simulink model "simModel2020"  (R2023b)
settings: Solver=ode4  StartTime=0  StopTime=360  FixedStep=0.01  RelTol=1e-3
values from neighbouring files (symbols this model uses):
  B747 =     [B747.mat]
undefined symbols (not defined in the file or in its folder): airport, APP, control, Curise, Earth, env, ft, m, navData, navParam, Newton, plotTrack, Raphson, s, TakeOff, WGS84
libraries: aerolibconvert2 x18, simulink x15, sharedtransform x4, aerolibfltsims x3, aerolibatmos2 x2, shared6dof x2, aerolibasang x2, dspsrcs4 x2, aerolibwind2 x2, aerolibanimutils x1, aerolibpropulsion2 x1, aerolibtransform2 x1
(part 1 of 6)
settings Model: Creator=yansui  LastModifiedBy=30359
settings SolverCC: AlgebraicLoopSolver=TrustRegion
settings DataIOCC: SaveFormat=StructureWithTime  ReturnWorkspaceOutputs=off
settings OptimizationCC: UseDivisionForNetSlopeComputation=UseDivisionForReciprocalsOfIntegersOnly  LifeSpan=inf
settings DebuggingCC: UnderspecifiedInitializationDetection=Classic  MergeDetectMultiDrivingBlocksExec=none  UnconnectedInputMsg=warning  UnconnectedOutputMsg=warning  UnconnectedLineMsg=warning  SFExecutionAtInitializationDiag=none  ArithmeticOperatorsInVariantConditions=warning
settings HardwareCC: ProdBitPerSizeT=32  ProdBitPerPtrDiffT=32  ProdWordSize=32  ProdHWDeviceType=Specified
settings ModelReferenceCC: EnableRefExpFcnMdlSchedulingChecks=on  PropagateSignalLabelsOutOfModel=off
settings SFSimCC: CustomCodeUndefinedFunction=UseInterfaceOnly
settings RTWCC: DLArmComputeVersion=19.05
settings CodeAppCC: StateflowObjectComments=on
settings SimscapeCC: SimscapeNormalizeSystem=off

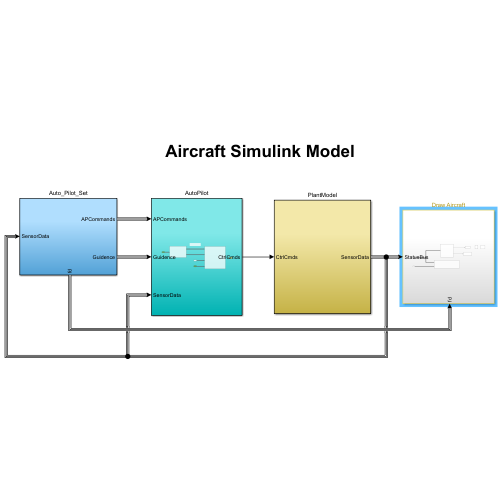
[thumbnail: Simulink's stored preview of the top-level diagram]
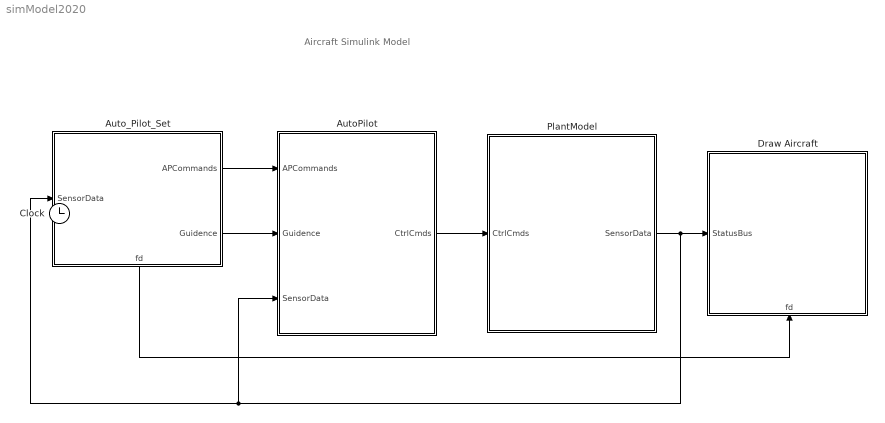
== system simModel2020 ==
  note: Aircraft Simulink Model
  AutoPilot : Subsystem
  Auto_Pilot_Set : Subsystem
      settings: PortSchema="{\"entries\":[{\"content\":{\"sides\":[{\"content\":{\"connectorIds\":[\"In1\"]},\"type\":\"ConnectorPlacement.EquallySpacedRectSide\",\"uuid\":\"ac12fa39-0519-46cb-816b-da74cf636ca7\"},{\"content\":{\"connectorIds\":[\"Out1\",\"Out2\"],\"side\":\"RIGHT\"},\"type\":\"ConnectorPlacement.EquallySpacedRectSide\",\"uuid\":\"cbf50b70-7502-46b3-9fdc-f239a08b8b7e\"},{\"content\":{\"connectorIds\":[],\"side\":\"TOP\"},\"type\":\"ConnectorPlacement.EquallySpacedRectSide\",\"uuid\":\"332bbf84-3788-4a39-9398-3a07aeea103a\"},{\"content\":{\"connectorIds\":[\"Out3\"],\"side\":\"BOTTOM\"},\"type\":\"ConnectorPlacement.EquallySpacedRectSide\",\"uuid\":\"7c0f671f-6fd4-43aa-82e5-0c8cee8639f5\"},{\"content\":{\"connectorIds\":[],\"side\":\"HIDDEN\"},\"type\":\"ConnectorPlacement.EquallySpacedRectSide\",\"uuid\":\"2f1a0ecd-686d-482d-b7d9-7339c0c9d807\"}]},\"type\":\"ConnectorPlacement.EquallySpacedConnector\",\"uuid\":\"bfc57a22-0ee0-4914-8111-1a37d4451974\"}],\"packageUris\":[\"http://schema.mathworks.com/mf0/Connector/R2020b\"],\"version\":\"1.0\"}"
  Draw Aircraft : Subsystem
      settings: PortSchema="{\"entries\":[{\"content\":{\"sides\":[{\"content\":{\"connectorIds\":[\"In1\"]},\"type\":\"ConnectorPlacement.EquallySpacedRectSide\",\"uuid\":\"f18468e1-33a6-4018-8fd5-26c86a421d63\"},{\"content\":{\"connectorIds\":[],\"side\":\"RIGHT\"},\"type\":\"ConnectorPlacement.EquallySpacedRectSide\",\"uuid\":\"f55cc71b-d18c-4aeb-b394-bdad06d8ea35\"},{\"content\":{\"connectorIds\":[],\"side\":\"TOP\"},\"type\":\"ConnectorPlacement.EquallySpacedRectSide\",\"uuid\":\"56c08431-7be0-4743-a300-4e3bf9f02124\"},{\"content\":{\"connectorIds\":[\"In2\"],\"side\":\"BOTTOM\"},\"type\":\"ConnectorPlacement.EquallySpacedRectSide\",\"uuid\":\"9c457df7-be2c-407c-bd8c-2d1e2b999c83\"},{\"content\":{\"connectorIds\":[],\"side\":\"HIDDEN\"},\"type\":\"ConnectorPlacement.EquallySpacedRectSide\",\"uuid\":\"89330191-b594-413f-b61d-27434e3fab37\"}]},\"type\":\"ConnectorPlacement.EquallySpacedConnector\",\"uuid\":\"9b92ccae-74d0-4af6-bd5d-a19e9caf359d\"}],\"packageUris\":[\"http://schema.mathworks.com/mf0/Connector/R2020b\"],\"version\":\"1.0\"}"
  PlantModel : Subsystem
  Clock : Clock
      settings: IOType=siggen
  wires:
  AutoPilot/1(CtrlCmds) -> PlantModel/1(CtrlCmds)
  Auto_Pilot_Set/2(Guidence) -> AutoPilot/2(Guidence)
  Auto_Pilot_Set/1(APCommands) -> AutoPilot/1(APCommands)
  PlantModel/1(SensorData) -> Auto_Pilot_Set/1(SensorData), AutoPilot/3(SensorData), Draw Aircraft/1(StatusBus)
  Auto_Pilot_Set/3(fd) -> Draw Aircraft/2(fd)

== system simModel2020/AutoPilot ==
  note: B747 Aircraft Controller
  APCommands : Inport
  Guidence : Inport  Port=2
  SensorData : Inport  Port=3  BusOutputAsStruct=on
  InnerLoopAutopilot : Subsystem  TreatAsAtomicUnit=on
  SensorFilter : Subsystem  TreatAsAtomicUnit=on
  CtrlCmds : Outport  BusOutputAsStruct=on
  wires:
  SensorData/1 -> SensorFilter/1(SensorData)
  SensorFilter/1(StateBus) -> InnerLoopAutopilot/1(StateBus)
  APCommands/1 -> InnerLoopAutopilot/3(APCommands)
  SensorFilter/2(Engine) -> InnerLoopAutopilot/2(Engine)
  Guidence/1 -> InnerLoopAutopilot/4(Guidence)
  InnerLoopAutopilot/1(CtrlCmds) -> CtrlCmds/1

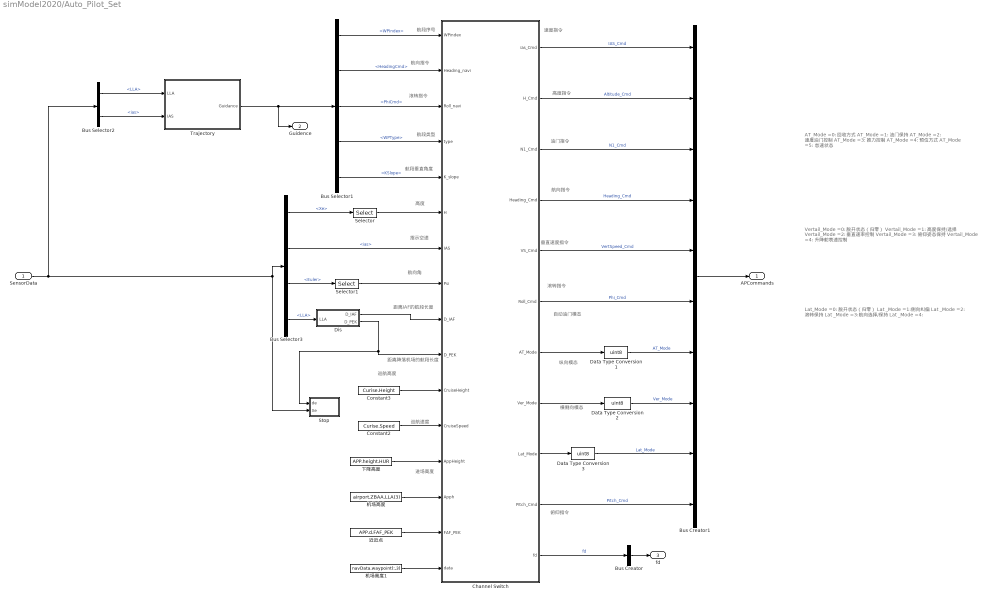
== system simModel2020/Auto_Pilot_Set ==
  note: 俯仰指令
  note: 横侧向模态
  note: 纵向模态
  note: 自动油门模态
  note: 滚转指令
  note: 垂直速度指令
  note: 航向指令
  note: 油门指令
  note: 高度指令
  note: 速度指令
  note: 航段序号
  note: 航向指令
  note: 滚转指令
  note: 航段类型
  note: 航段垂直角度
  note: 高度
  note: 指示空速
  note: 航向角
  note: 进场高度
  note: 巡航速度
  note: 巡航高度
  note: Lat_Mode =0: 脱开状态（归零）
      | Lat _Mode =1:侧向纠偏
      | Lat _Mode =2: 滚转保持
      | Lat _Mode =3:航向选择/保持
      | Lat _Mode =4:
  note: Vertail_Mode =0: 脱开状态（归零）
      | Vertail_Mode =1: 高度保持/选择
      | Vertail_Mode =2: 垂直速率控制
      | Vertail_Mode =3: 俯仰姿态保持
      | Vertail_Mode =4: 升降舵表速控制
  note: AT_Mode =0: 回收方式
      | AT_Mode =1: 油门保持
      | AT_Mode =2: 速度油门控制
      | AT_Mode =3: 推力控制
      | AT_Mode =4: 预位方式
      | AT_Mode =5: 怠速状态
  note: 距离IAF的航段长度
  note: 距离降落机场的航段长度
  SensorData : Inport
  Bus Creator : BusCreator  Inputs=1
  Bus Creator1 : BusCreator  Inputs=10
  Bus Selector1 : BusSelector  OutputSignals=WPIndex,HeadingCmd,PhiCmd,WPType,KSlope
  Bus Selector2 : BusSelector  OutputSignals=LLA,ias
  Bus Selector3 : BusSelector  OutputSignals=Xe,ias,Euler,LLA
  Channel Switch : Stateflow chart  TreatAsAtomicUnit=on
  Constant2 : Constant  Value=Curise.Speed
  Constant3 : Constant  Value=Curise.Height
  Data Type Conversion1 : DataTypeConversion  OutDataTypeStr=uint8  SaturateOnIntegerOverflow=off  RndMeth=Floor
  Data Type Conversion2 : DataTypeConversion  OutDataTypeStr=uint8  SaturateOnIntegerOverflow=off  RndMeth=Floor
  Data Type Conversion3 : DataTypeConversion  OutDataTypeStr=uint8  SaturateOnIntegerOverflow=off  RndMeth=Floor
  Dis : Subsystem
  Selector : Selector  InputPortWidth=3  IndexOptions=Index vector (dialog)  Indices=[3]  OutputSizes=1
  Selector1 : Selector  InputPortWidth=3  IndexOptions=Index vector (dialog)  Indices=[3]  OutputSizes=1
  Stop : Subsystem
  Trajectory : Subsystem
  下降高度 : Constant  Value=APP.height.HUR
  机场高度 : Constant  Value=airport.ZBAA.LLA(3)
  机场高度1 : Constant  Value=navData.waypoint(:,3)
  近近点 : Constant  Value=APP.d.FAF_PEK
  APCommands : Outport
  Guidence : Outport  Port=2
  fd : Outport  Port=3
  wires:
  Channel Switch/3(N1_Cmd) -> Bus Creator1/3  "N1_Cmd"
  Channel Switch/1(ias_Cmd) -> Bus Creator1/1  "IAS_Cmd"
  Channel Switch/5(VS_Cmd) -> Bus Creator1/5  "VertSpeed_Cmd"
  Channel Switch/2(H_Cmd) -> Bus Creator1/2  "Altitude_Cmd"
  Channel Switch/4(Heading_Cmd) -> Bus Creator1/4  "Heading_Cmd"
  Channel Switch/6(Roll_Cmd) -> Bus Creator1/6  "Phi_Cmd"
  Data Type Conversion3/1 -> Bus Creator1/9  "Lat_Mode"
  Data Type Conversion2/1 -> Bus Creator1/8  "Ver_Mode"
  Data Type Conversion1/1 -> Bus Creator1/7  "AT_Mode"
  Bus Selector3/4 -> Dis/1(LLA)  "<LLA>"
  Dis/1(D_IAF) -> Channel Switch/9(D_IAF)
  Dis/2(D_PEK) -> Stop/1(de), Channel Switch/10(D_PEK)
  Constant3/1 -> Channel Switch/11(CruiseHeight)
  Constant2/1 -> Channel Switch/12(CruiseSpeed)
  下降高度/1 -> Channel Switch/13(AppHeight)
  Bus Selector3/2 -> Channel Switch/7(IAS)  "<ias>"
  Bus Selector3/1 -> Selector/1  "<Xe>"
  Selector/1 -> Channel Switch/6(H)
  Bus Creator1/1 -> APCommands/1
  SensorData/1 -> Bus Selector2/1, Stop/2(Xe), Bus Selector3/1
  Channel Switch/7(AT_Mode) -> Data Type Conversion1/1
  Channel Switch/8(Ver_Mode) -> Data Type Conversion2/1
  Channel Switch/9(Lat_Mode) -> Data Type Conversion3/1
  Trajectory/1(Guidance) -> Guidence/1, Bus Selector1/1
  Bus Selector1/2 -> Channel Switch/2(Heading_navi)  "<HeadingCmd>"
  Bus Selector1/3 -> Channel Switch/3(Roll_navi)  "<PhiCmd>"
  Bus Selector1/4 -> Channel Switch/4(type)  "<WPType>"
  Bus Selector1/5 -> Channel Switch/5(K_slope)  "<KSlope>"
  Bus Selector2/1 -> Trajectory/1(LLA)  "<LLA>"
  Bus Selector2/2 -> Trajectory/2(IAS)  "<ias>"
  Bus Selector1/1 -> Channel Switch/1(WPindex)  "<WPIndex>"
  Bus Selector3/3 -> Selector1/1  "<Euler>"
  Selector1/1 -> Channel Switch/8(Psi)
  Channel Switch/10(Pitch_Cmd) -> Bus Creator1/10  "Pitch_Cmd"
  机场高度/1 -> Channel Switch/14(Apph)
  近近点/1 -> Channel Switch/15(FAF_PEK)
  机场高度1/1 -> Channel Switch/16(data)
  Channel Switch/11(fd) -> Bus Creator/1  "fd"
  Bus Creator/1 -> fd/1

== system simModel2020/Draw Aircraft ==
  StatusBus : Inport
  fd : Inport  Port=2
  DataOut : Subsystem
  DataToFlightgear : Subsystem
  FlightGear : Subsystem
  Generate Run Script1 : aerolibfltsims/Generate Run Script  Architecture=Win64  dataFlow=Send  GeometryModelName=f15c  AirportId=ZUUU  RunwayId=20  InitialAltitude=0  InitialHeading=200  OffsetDistance=0  OffsetAzimuth=0  InstallScenery=on  DisableShaders=off  OriginAddress=127.0.0.1  DestinationPort=5502  OriginPort=5505  LocalAddress=127.0.0.1  OutputFileName=runfg.bat  FlightGearBaseDirectory=D:\MATLAB\FlightGear 2020.3
  Interpreted MATLAB Function1 : MATLABFcn  MATLABFcn=plotTrack(u)  OutputDimensions=0  Output1D=off
  Simulation Pace : aerolibanimutils/Simulation Pace  SimulationPace=100  SleepMode=MATLAB Thread  OutputPaceError=off  SampleTime=B747.sampleTime
      settings: AttributesFormatString=%<SimulationPace> sec/sec
  wires:
  StatusBus/1 -> DataToFlightgear/1(In1), DataOut/1(In)
  DataToFlightgear/1(Out1) -> Interpreted MATLAB Function1/1
  DataToFlightgear/2(Out2) -> FlightGear/1(In1)
  fd/1 -> DataOut/2(fd)

== system simModel2020/PlantModel ==
  CtrlCmds : Inport  SampleTime=B747.sampleTime
  Actuator Model : Subsystem
  "Air Sensor " : Subsystem
  B747 Dynamics动力学参数计算 : Subsystem
  Constant2 : Constant  Value=0
  FlightSwitchModel : Subsystem
  Sensor Model : Subsystem
  Wind Model : Subsystem
  WindSelect : Constant  Value=0
  SensorData : Outport
  wires:
  B747 Dynamics动力学参数计算/2(AirData) -> "Air Sensor "/2(AirData)
  B747 Dynamics动力学参数计算/1(B747 State) -> Wind Model/1(uavState), "Air Sensor "/1(B747 State), Sensor Model/1(B747 State)
  "Air Sensor "/2(Rho) -> B747 Dynamics动力学参数计算/3(Rho)  "rho"
  Actuator Model/1(ctrlSurfaces) -> Sensor Model/5(CtrlSurfaces), B747 Dynamics动力学参数计算/2(CtrlSurfaces)
  "Air Sensor "/1(AirSensorData) -> Sensor Model/3(AirSensorData)
  Wind Model/1(Wind_e) -> B747 Dynamics动力学参数计算/1(Wind_e)
  B747 Dynamics动力学参数计算/3(Engine) -> Sensor Model/4(Engine)
  "Air Sensor "/3(Speed of Sound) -> B747 Dynamics动力学参数计算/4(Speed of Sound)
  Constant2/1 -> B747 Dynamics动力学参数计算/5(Deviation On)
  Sensor Model/1(SensorData) -> SensorData/1
  CtrlCmds/1 -> FlightSwitchModel/1(CtrlCmds)
  FlightSwitchModel/1(ctrlcmds) -> Actuator Model/1(ctrlcmds)
  B747 Dynamics动力学参数计算/4(Wind) -> Sensor Model/2(Wind)
  WindSelect/1 -> Wind Model/2(Wind On)

== system simModel2020/AutoPilot/InnerLoopAutopilot ==
  note: 纵向
  note: 横侧向
  StateBus : Inport
  Engine : Inport  Port=2
  APCommands : Inport  Port=3
  Guidence : Inport  Port=4
  Bus Selector : BusSelector  OutputSignals=N1
  Constant2 : Constant  Value=0  OutDataTypeStr=Inherit: Inherit via back propagation
  Latitudinal Channel维度通道 : Subsystem
  Longitudinal Channel经度通道 : Subsystem  TreatAsAtomicUnit=on
  Mux : Mux  Inputs=5
  CtrlCmds : Outport
  wires:
  APCommands/1 -> Latitudinal Channel维度通道/1(APCommands), Longitudinal Channel经度通道/3(APCommands)
  StateBus/1 -> Latitudinal Channel维度通道/2(apStatus), Longitudinal Channel经度通道/1(StatusBus)
  Engine/1 -> Bus Selector/1
  Bus Selector/1 -> Longitudinal Channel经度通道/2(N1)  "<N1>"
  Constant2/1 -> Mux/5  "flapCmd襟翼"
  Guidence/1 -> Latitudinal Channel维度通道/3(Guidence)
  Longitudinal Channel经度通道/1(dE) -> Mux/1  "elevatorCmd升降舵"
  Longitudinal Channel经度通道/2(dT) -> Mux/2  "throttleCmd油门"
  Latitudinal Channel维度通道/1(dA) -> Mux/3  "aileronCmd副翼"
  Latitudinal Channel维度通道/2(dR) -> Mux/4  "rudderCmd方向舵"
  Mux/1 -> CtrlCmds/1

== system simModel2020/AutoPilot/SensorFilter ==
  SensorData : Inport
  Bus Creator : BusCreator  Inputs=2
  Bus Creator1 : BusCreator  Inputs=12
  Bus Selector : BusSelector  OutputSignals=Euler,Ab,pqr,q,static,OAT,alpha,beta,Xe,Ve,ias,IsGround,N1,FQ
  StateBus : Outport
  Engine : Outport  Port=2
  wires:
  Bus Creator/1 -> Engine/1
  Bus Creator1/1 -> StateBus/1
  Bus Selector/14 -> Bus Creator/2  "<FQ>"
  SensorData/1 -> Bus Selector/1
  Bus Selector/13 -> Bus Creator/1  "<N1>"
  Bus Selector/10 -> Bus Creator1/10  "<Ve>"
  Bus Selector/8 -> Bus Creator1/8  "<beta>"
  Bus Selector/6 -> Bus Creator1/6  "<OAT>"
  Bus Selector/7 -> Bus Creator1/7  "<alpha>"
  Bus Selector/9 -> Bus Creator1/9  "<Xe>"
  Bus Selector/5 -> Bus Creator1/5  "<static>"
  Bus Selector/3 -> Bus Creator1/3  "<pqr>"
  Bus Selector/4 -> Bus Creator1/4  "<q>"
  Bus Selector/2 -> Bus Creator1/2  "<Ab>"
  Bus Selector/1 -> Bus Creator1/1  "<Euler>"
  Bus Selector/11 -> Bus Creator1/11  "<ias>"
  Bus Selector/12 -> Bus Creator1/12  "<IsGround>"

== system simModel2020/Auto_Pilot_Set/Dis ==
  note: 距离降落机场的航段长度
  note: 距离IAF的航段长度
  note: 导航参数
  note: 着陆机场位置
  note: IAF位置
  LLA : Inport
  Constant5 : Constant  Value=APP.pos.IAF
  Constant6 : Constant  Value=APP.pos.PEK
  Constant7 : Constant  Value=navParam.FQParam
  MATLAB Function2 : MATLAB Function  TreatAsAtomicUnit=on
  D_IAF : Outport
  D_PEK : Outport  Port=2
  wires:
  LLA/1 -> MATLAB Function2/1(LLA)
  MATLAB Function2/2(D_PEK) -> D_PEK/1
  MATLAB Function2/1(D_IAF) -> D_IAF/1
  Constant6/1 -> MATLAB Function2/3(PEK)
  Constant7/1 -> MATLAB Function2/4(FQParam)
  Constant5/1 -> MATLAB Function2/2(IAF)

== system simModel2020/Auto_Pilot_Set/Stop ==
  de : Inport
  Xe : Inport  Port=2
  Bus Selector4 : BusSelector  OutputSignals=Xe
  Compare To Constant : simulink/Logic and Bit Operations/Compare To Constant  relop=<=  const=airport.ZBAA.LLA(end)  OutDataTypeStr=boolean
  Compare To Constant1 : simulink/Logic and Bit Operations/Compare To Constant  relop=<=  const=100  OutDataTypeStr=boolean
  Logical Operator1 : Logic  Operator=OR  AllPortsSameDT=off  OutDataTypeStr=boolean
  Selector2 : Selector  InputPortWidth=3  IndexOptions=Index vector (dialog)  Indices=[3]  OutputSizes=1
  Stop Simulation : Stop
  wires:
  Bus Selector4/1 -> Selector2/1  "<Xe>"
  Compare To Constant/1 -> Logical Operator1/2
  Compare To Constant1/1 -> Logical Operator1/1
  Selector2/1 -> Compare To Constant/1
  de/1 -> Compare To Constant1/1
  Logical Operator1/1 -> Stop Simulation/1
  Xe/1 -> Bus Selector4/1

== system simModel2020/Auto_Pilot_Set/Trajectory ==
  note: 滚转指令
  note: 航段方位角
  note: 航段间垂直角度
  note: 航路点高度
  note: 重力加速度
  note: 圆弧初始位置P1，P1->P2航向，圆心位置，高度，转弯方向，转弯半径
  note: 转弯方向
  note: 航段类型
  note: 航段序号
  note: 导航计算参数
  note: 转弯圆心位置、航段距离、转向、航向角
  note: 航段纬经高、长度、方位角
  note: 初始航段：直线
  note: 航段类型 0圆弧 1直线
      | 转弯方向 -1 左转 1 右转 0直线
  LLA : Inport
  IAS : Inport  Port=2
  Bus Creator1 : BusCreator  Inputs=6
  Clock : Clock
  Constant : Constant  Value=navData.InitialIndex
  Constant1 : Constant  Value=navData.FlightLineSeg
  Constant2 : Constant  Value=navData.FlightCircleSeg
  Constant3 : Constant  Value=navParam.FQParam
  Constant4 : Constant  Value=navData.waypoint(:,3)
  Constant5 : Constant  Value=navData.FlightCircleP0
  Constant7 : Constant  Value=navParam.g
  Display : Display
  Display1 : Display
  Display3 : Display
  MATLAB Function : MATLAB Function  TreatAsAtomicUnit=on
  MATLAB Function1 : MATLAB Function  TreatAsAtomicUnit=on
  Subsystem : Subsystem
  Guidance : Outport
  wires:
  Constant/1 -> MATLAB Function/2(InitialIndex)
  Clock/1 -> MATLAB Function/1(t)
  Constant1/1 -> MATLAB Function1/3(FlightLineSeg), MATLAB Function/3(FlightLineSeg)
  Constant2/1 -> MATLAB Function/4(FlightCircleSeg)
  Constant3/1 -> MATLAB Function/5(FQParam), MATLAB Function1/4(FQParam)
  MATLAB Function/1(WPIndex) -> Bus Creator1/1, MATLAB Function1/1(WPIndex), Display/1  "WPIndex"
  MATLAB Function/2(WPType) -> Bus Creator1/2, Display1/1, MATLAB Function1/2(WPType)  "WPType"
  LLA/1 -> MATLAB Function/6(LLA), MATLAB Function1/5(LLA)
  Bus Creator1/1 -> Guidance/1
  MATLAB Function1/1(LatDistance) -> Subsystem/1(In1), Bus Creator1/3  "LatDistance"
  Subsystem/1(Out1) -> Bus Creator1/4  "PhiCmd"
  MATLAB Function1/3(HeadingCmd) -> Bus Creator1/5  "HeadingCmd"
  MATLAB Function1/4(KSlope) -> Bus Creator1/6  "KSlope"
  IAS/1 -> MATLAB Function1/6(IAS)
  Constant5/1 -> MATLAB Function1/7(FlightCircleP0)
  Constant7/1 -> MATLAB Function1/8(g)
  MATLAB Function/3(Turn) -> Display3/1  "Turn"
  Constant4/1 -> MATLAB Function1/9(WayPointAlt)
  MATLAB Function1/2(Phig) -> Subsystem/2(In2)  "PhiCmd"

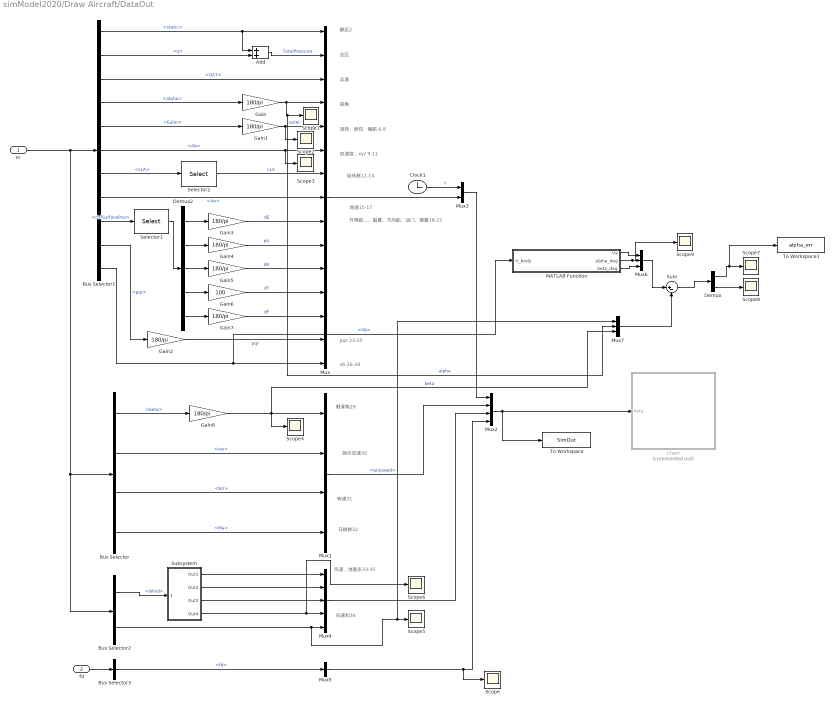
== system simModel2020/Draw Aircraft/DataOut ==
  note: 风速和36
  note: 马赫数32
  note: 转速31
  note: 指示空速30
  note: 侧滑角29
  note: 升降舵、副翼、方向舵、油门、襟翼18-22
  note: vb 26-28
  note: pqr 23-25
  note: 地速15-17
  note: 经纬高12-14
  note: 加速度，xyz 9-11
  note: 滚转、俯仰、偏航 6-8
  note: 迎角
  note: 总温
  note: 总压
  note: 静压2
  note: 风速，地面系33-35
  In : Inport
  fd : Inport  Port=2
  Add : Sum
  Bus Selector : BusSelector  OutputSignals=beta,ias,N1,Ma
  Bus Selector1 : BusSelector  OutputSignals=static,q,OAT,alpha,Euler,Ab,LLA,Ve,ctrlSurfacePos,pqr,Vb
  Bus Selector2 : BusSelector  OutputSignals=Wind,airpseed
  Bus Selector3 : BusSelector  OutputSignals=fd
  Chart : Stateflow chart  Commented=on  TreatAsAtomicUnit=on
  Clock1 : Clock
  Demux : Demux  Outputs=[1 2]
  Demux2 : Demux  Outputs=5
  Gain{,1..5,7..8} (8 alike) : Gain  Gain=180/pi
  Gain6 : Gain  Gain=100
  MATLAB Function : MATLAB Function  TreatAsAtomicUnit=on
  Mux : Mux  Inputs=15
  Mux1 : Mux
  Mux2 : Mux
  Mux3 : Mux  Inputs=2
  Mux4 : Mux  Inputs=5
  Mux5 : Mux  Inputs=1
  Mux6 : Mux  Inputs=3
  Mux7 : Mux  Inputs=3
  Scope{,1..9} (10 alike) : Scope
  Selector1 : Selector  InputPortWidth=5  IndexOptions=Index vector (dialog)  Indices=[1 3 4 2 5]  OutputSizes=1
  Selector2 : Selector  InputPortWidth=3  IndexOptions=Index vector (dialog)  Indices=[2 1 3 ]  OutputSizes=1
  Subsystem : Subsystem
  Sum : Sum  Inputs=|+-
  To Workspace : ToWorkspace  VariableName=SimOut  SampleTime=-1
      settings: Save2DSignal=2-D array (concatenate along first dimension)
  To Workspace1 : ToWorkspace  VariableName=alpha_err  SaveFormat=Timeseries  SampleTime=-1
  wires:
  Demux2/1 -> Gain3/1
  Bus Selector1/11 -> MATLAB Function/1(V_body), Mux/15  "<Vb>"
  Bus Selector1/7 -> Selector2/1  "<LLA>"
  Gain/1 -> Mux7/2, Scope1/1, Mux/4  "alpha"
  Demux2/3 -> Gain5/1
  Bus Selector1/6 -> Mux/6, Scope3/1  "<Ab>"
  Bus Selector1/5 -> Gain1/1  "<Euler>"
  Selector2/1 -> Mux/7  "LLA"
  Bus Selector1/10 -> Gain2/1  "<pqr>"
  Demux2/5 -> Gain7/1
  Bus Selector1/2 -> Add/2  "<q>"
  Gain7/1 -> Mux/13  "dF"
  Mux/1 -> Mux3/2
  Gain5/1 -> Mux/11  "dR"
  Bus Selector1/3 -> Mux/3  "<OAT>"
  Bus Selector1/4 -> Gain/1  "<alpha>"
  In/1 -> Bus Selector2/1, Bus Selector/1, Bus Selector1/1
  Demux2/2 -> Gain4/1
  Mux3/1 -> Mux2/1
  Gain2/1 -> Mux/14  "pqr"
  Gain3/1 -> Mux/9  "dE"
  Bus Selector1/9 -> Selector1/1  "<ctrlSurfacePos>"
  Selector1/1 -> Demux2/1
  Add/1 -> Mux/2  "TotalPressure"
  Clock1/1 -> Mux3/1  "t"
  Bus Selector1/1 -> Add/1, Mux/1  "<static>"
  Gain6/1 -> Mux/12  "dT"
  Gain1/1 -> Scope2/1, Mux/5  "euler"
  Demux2/4 -> Gain6/1
  Bus Selector1/8 -> Mux/8  "<Ve>"
  Gain4/1 -> Mux/10  "dA"
  Bus Selector/2 -> Mux1/2  "<ias>"
  Bus Selector/1 -> Gain8/1  "<beta>"
  Bus Selector/3 -> Mux1/3  "<N1>"
  Bus Selector/4 -> Mux1/4  "<Ma>"
  Gain8/1 -> Mux7/3, Scope4/1, Mux1/1  "beta"
  Mux1/1 -> Mux2/2
  Mux2/1 -> Chart/1(data), To Workspace/1
  Mux4/1 -> Mux2/3
  Bus Selector2/2 -> Mux7/1, Scope5/1, Mux4/5  "<airpseed>"
  Bus Selector2/1 -> Subsystem/1(<Wind>)  "<Wind>"
  Subsystem/1(Out1) -> Mux4/1
  Subsystem/2(Out2) -> Mux4/2
  Subsystem/3(Out3) -> Mux4/3
  Subsystem/4(Out4) -> Scope6/1, Mux4/4
  fd/1 -> Bus Selector3/1
  Bus Selector3/1 -> Mux5/1  "<fd>"
  Mux5/1 -> Scope/1, Mux2/4
  MATLAB Function/1(Va) -> Mux6/1
  MATLAB Function/2(alpha_deg) -> Scope9/1, Mux6/2
  MATLAB Function/3(beta_deg) -> Mux6/3
  Mux6/1 -> Sum/1
  Mux7/1 -> Sum/2
  Sum/1 -> Demux/1
  Demux/1 -> To Workspace1/1, Scope7/1
  Demux/2 -> Scope8/1

== system simModel2020/Draw Aircraft/DataToFlightgear ==
  note: 经纬高 滚转 俯仰 偏航
  In1 : Inport
  Angle Conversion1 : aerolibconvert2/Angle Conversion  IU=rad  OU=deg
  Angle Conversion2 : aerolibconvert2/Angle Conversion  IU=rad  OU=deg
  Angle Conversion3 : aerolibconvert2/Angle Conversion  IU=rad  OU=deg
  Bus Selector : BusSelector  OutputSignals=LLA,Euler,ias,airpseed,alpha,beta
  Clock : Clock
  Constant : Constant  Commented=on  Value=4000
  Data Type Conversion9 : DataTypeConversion  OutDataTypeStr=double  SaturateOnIntegerOverflow=off  RndMeth=Floor
  Demux : Demux  Outputs=[2,1]
  Demux1 : Demux  Outputs=3
  Mux1 : Mux  Inputs=2
  Mux2 : Mux  Inputs=3
  Rate Transition1 : RateTransition  OutPortSampleTime=1
  Scope : Scope  NumInputPorts=8
  Selector : Selector  InputPortWidth=2  IndexOptions=Index vector (dialog)  Indices=[2 1]  OutputSizes=1
  Sum : Sum  Inputs=|+-
  Out1 : Outport
  Out2 : Outport  Port=2
  wires:
  Demux/2 -> Sum/1, Scope/1  "<gps_h>"
  Data Type Conversion9/1 -> Mux2/3
  Angle Conversion2/1 -> Scope/8  "beta"
  Mux1/1 -> Rate Transition1/1
  Selector/1 -> Mux2/1
  Bus Selector/2 -> Angle Conversion3/1, Data Type Conversion9/1  "<Euler>"
  Bus Selector/6 -> Angle Conversion2/1  "<beta>"
  Demux1/2 -> Scope/3  "theta"
  Clock/1 -> Mux1/2
  Angle Conversion3/1 -> Demux1/1
  Mux2/1 -> Out2/1
  Demux1/1 -> Scope/2  "phi"
  Bus Selector/3 -> Scope/5  "<ias>"
  Demux1/3 -> Scope/4  "Psi"
  Bus Selector/1 -> Demux/1, Mux1/1  "<LLA>"
  Bus Selector/4 -> Scope/6  "<airpseed>"
  Demux/1 -> Selector/1
  Angle Conversion1/1 -> Scope/7  "alpha"
  Bus Selector/5 -> Angle Conversion1/1  "<alpha>"
  In1/1 -> Bus Selector/1
  Rate Transition1/1 -> Out1/1
  Sum/1 -> Mux2/2
  Constant/1 -> Sum/2

== system simModel2020/Draw Aircraft/FlightGear ==
  In1 : Inport
  Angle Conversion : Subsystem
  Angle Conversion1 : Subsystem
  Demux : Demux  Outputs=6
  Pack net_fdm Packet for FlightGear1 : aerolibfltsims/Pack net_fdm Packet for FlightGear  FlightGearVersion=v2019.1  ShowPositionAttitudeInputs=on  ShowVelocityAccelerationInputs=off  ShowControlSurfacePositionInputs=off  ShowEngineFuelInputs=off  ShowLandingGearInputs=off  ShowEnvironmentInputs=off  SampleTime=-1  packetVersion=24
  Rate Transition : RateTransition  Integrity=off  Deterministic=off
  Send net_fdm Packet to FlightGear : aerolibfltsims/Send net_fdm Packet to FlightGear  DestinationIpAddress=127.0.0.1  DestinationPort=5502  LocalIpPort=-1  varLen=off  SampleTime=-1
  toSingle1 : DataTypeConversion  OutDataTypeStr=single  SaturateOnIntegerOverflow=off  RndMeth=Floor
  toSingle2 : DataTypeConversion  OutDataTypeStr=single  SaturateOnIntegerOverflow=off  RndMeth=Floor
  toSingle3 : DataTypeConversion  OutDataTypeStr=single  SaturateOnIntegerOverflow=off  RndMeth=Floor
  wires:
  Angle Conversion/1(out) -> Pack net_fdm Packet for FlightGear1/1
  toSingle2/1 -> Pack net_fdm Packet for FlightGear1/5
  toSingle1/1 -> Pack net_fdm Packet for FlightGear1/4
  Demux/3 -> Pack net_fdm Packet for FlightGear1/3
  In1/1 -> Rate Transition/1
  Demux/1 -> Angle Conversion/1(in)
  Rate Transition/1 -> Demux/1
  Angle Conversion1/1(out) -> Pack net_fdm Packet for FlightGear1/2
  Demux/2 -> Angle Conversion1/1(in)
  toSingle3/1 -> Pack net_fdm Packet for FlightGear1/6
  Demux/4 -> toSingle1/1
  Demux/5 -> toSingle2/1
  Demux/6 -> toSingle3/1
  Pack net_fdm Packet for FlightGear1/1 -> Send net_fdm Packet to FlightGear/1

== system simModel2020/PlantModel/Actuator Model ==
  ctrlcmds : Inport
  Bus Creator1 : BusCreator  Inputs=5
  Data Type Conversion{1..4,7} (5 alike) : DataTypeConversion  OutDataTypeStr=double  SaturateOnIntegerOverflow=off  RndMeth=Floor
  Demux : Demux  Outputs=5
  Linear Second Order Actuators : Subsystem  mask(LinearSecondOrderActuator){wn_fin=35, z_fin=0.75, fin_act_0=0, fin_act_vel=0}
      mask prompts: wn_fin "aeroblks:aeroblkactuator:blockLinearSecondOrderActuatorParamNaturalfrequency"; z_fin "aeroblks:aeroblkactuator:blockLinearSecondOrderActuatorParamDampingratio"; fin_act_0 "aeroblks:aeroblkactuator:blockLinearSecondOrderActuatorParamInitialposition"; fin_act_vel "aeroblks:aeroblkactuator:blockLinearSecondOrderActuatorParamInitialvelocity"
      mask help: aeroblks:aeroblkactuator:blockLinearSecondOrderActuatorDesc
      mask init:
      | aeroicon('aeroblkactuator')
      settings: AttributesFormatString=|
      | Nat Freq => %<wn_fin>
      | Damping => %<z_fin>
      mask Help: eval('asbhelp');
      mask Display:
      | port_label('input',1,'A_{demand}','texmode','on');
      | port_label('output',1,'A_{actual}','texmode','on');
  Linear Second-Order Actuator1 : Subsystem  mask(LinearSecondOrderActuator){wn_fin=35, z_fin=0.75, fin_act_0=0, fin_act_vel=0}
      mask prompts: wn_fin "aeroblks:aeroblkactuator:blockLinearSecondOrderActuatorParamNaturalfrequency"; z_fin "aeroblks:aeroblkactuator:blockLinearSecondOrderActuatorParamDampingratio"; fin_act_0 "aeroblks:aeroblkactuator:blockLinearSecondOrderActuatorParamInitialposition"; fin_act_vel "aeroblks:aeroblkactuator:blockLinearSecondOrderActuatorParamInitialvelocity"
      mask help: aeroblks:aeroblkactuator:blockLinearSecondOrderActuatorDesc
      mask init:
      | aeroicon('aeroblkactuator')
      mask Help: eval('asbhelp');
      mask Display:
      | port_label('input',1,'A_{demand}','texmode','on');
      | port_label('output',1,'A_{actual}','texmode','on');
  Linear Second-Order Actuator2 : Subsystem  mask(LinearSecondOrderActuator){wn_fin=35, z_fin=0.75, fin_act_0=0, fin_act_vel=0}
      mask prompts: wn_fin "aeroblks:aeroblkactuator:blockLinearSecondOrderActuatorParamNaturalfrequency"; z_fin "aeroblks:aeroblkactuator:blockLinearSecondOrderActuatorParamDampingratio"; fin_act_0 "aeroblks:aeroblkactuator:blockLinearSecondOrderActuatorParamInitialposition"; fin_act_vel "aeroblks:aeroblkactuator:blockLinearSecondOrderActuatorParamInitialvelocity"
      mask help: aeroblks:aeroblkactuator:blockLinearSecondOrderActuatorDesc
      mask init:
      | aeroicon('aeroblkactuator')
      mask Help: eval('asbhelp');
      mask Display:
      | port_label('input',1,'A_{demand}','texmode','on');
      | port_label('output',1,'A_{actual}','texmode','on');
  Linear Second-Order Actuator3 : Subsystem  mask(LinearSecondOrderActuator){wn_fin=35, z_fin=0.75, fin_act_0=0, fin_act_vel=0}
      mask prompts: wn_fin "aeroblks:aeroblkactuator:blockLinearSecondOrderActuatorParamNaturalfrequency"; z_fin "aeroblks:aeroblkactuator:blockLinearSecondOrderActuatorParamDampingratio"; fin_act_0 "aeroblks:aeroblkactuator:blockLinearSecondOrderActuatorParamInitialposition"; fin_act_vel "aeroblks:aeroblkactuator:blockLinearSecondOrderActuatorParamInitialvelocity"
      mask help: aeroblks:aeroblkactuator:blockLinearSecondOrderActuatorDesc
      mask init:
      | aeroicon('aeroblkactuator')
      mask Help: eval('asbhelp');
      mask Display:
      | port_label('input',1,'A_{demand}','texmode','on');
      | port_label('output',1,'A_{actual}','texmode','on');
  Linear Second-Order Actuator4 : Subsystem  mask(LinearSecondOrderActuator){wn_fin=35, z_fin=0.75, fin_act_0=0, fin_act_vel=0}
      mask prompts: wn_fin "aeroblks:aeroblkactuator:blockLinearSecondOrderActuatorParamNaturalfrequency"; z_fin "aeroblks:aeroblkactuator:blockLinearSecondOrderActuatorParamDampingratio"; fin_act_0 "aeroblks:aeroblkactuator:blockLinearSecondOrderActuatorParamInitialposition"; fin_act_vel "aeroblks:aeroblkactuator:blockLinearSecondOrderActuatorParamInitialvelocity"
      mask help: aeroblks:aeroblkactuator:blockLinearSecondOrderActuatorDesc
      mask init:
      | aeroicon('aeroblkactuator')
      mask Help: eval('asbhelp');
      mask Display:
      | port_label('input',1,'A_{demand}','texmode','on');
      | port_label('output',1,'A_{actual}','texmode','on');
  Rate Transition{,1..4} (5 alike) : RateTransition  OutPortSampleTime=0
  ctrlSurfaces : Outport
  wires:
  Rate Transition4/1 -> Data Type Conversion4/1
  Rate Transition3/1 -> Data Type Conversion3/1
  Rate Transition2/1 -> Data Type Conversion2/1
  Rate Transition1/1 -> Data Type Conversion1/1
  Rate Transition/1 -> Data Type Conversion7/1
  ctrlcmds/1 -> Demux/1
  Data Type Conversion7/1 -> Linear Second-Order Actuator4/1(Ac_dem)
  Data Type Conversion1/1 -> Linear Second-Order Actuator3/1(Ac_dem)
  Data Type Conversion2/1 -> Linear Second-Order Actuator2/1(Ac_dem)
  Data Type Conversion3/1 -> Linear Second-Order Actuator1/1(Ac_dem)
  Data Type Conversion4/1 -> Linear Second Order Actuators/1(Ac_dem)
  Bus Creator1/1 -> ctrlSurfaces/1
  Demux/1 -> Rate Transition/1
  Demux/4 -> Rate Transition3/1
  Demux/5 -> Rate Transition4/1
  Demux/3 -> Rate Transition2/1
  Demux/2 -> Rate Transition1/1
  Linear Second-Order Actuator4/1(Ac_ac) -> Bus Creator1/1  "dE"
  Linear Second-Order Actuator3/1(Ac_ac) -> Bus Creator1/2  "dT"
  Linear Second-Order Actuator2/1(Ac_ac) -> Bus Creator1/3  "dA"
  Linear Second-Order Actuator1/1(Ac_ac) -> Bus Creator1/4  "dR"
  Linear Second Order Actuators/1(Ac_ac) -> Bus Creator1/5  "dF"

== system simModel2020/PlantModel/Air Sensor  ==
  note: ias = V
  B747 State : Inport
  AirData : Inport  Port=2
  Bus Creator : BusCreator  Inputs=9
  Bus Selector1 : BusSelector  OutputSignals=airpseed,q,alpha,beta,Ma
  Bus Selector3 : BusSelector  OutputSignals=Xe
  Gain : Gain  Gain=-1
      settings: AttributesFormatString=Z to Alt
  Gain1 : Gain
  Get Z : Selector  InputPortWidth=3  IndexOptions=Index vector (dialog)  Indices=[3]  OutputSizes=[(-2)]
  ISA Atmosphere Model : aerolibatmos2/ISA Atmosphere Model  useExtended=off  action=Warning  custom=on  viscosityOut=off  g=env.ISA_g  gamma=1.4  R=env.ISA_R  L=env.ISA_lapse  h_trop=11000  h_strat=50000  rho0=env.ISA_rho0  P0=env.ISA_P0  T0=env.ISA_T0  h0=0
  Temperature Conversion : aerolibconvert2/Temperature Conversion  IU=K  OU=C
  AirSensorData : Outport
  Rho : Outport  Port=2
  Speed of Sound : Outport  Port=3
  wires:
  Bus Selector3/1 -> Get Z/1  "<Xe>"
  Temperature Conversion/1 -> Bus Creator/1  "OAT"
  Bus Selector1/1 -> Gain1/1, Bus Creator/4  "<airpseed>"
  Bus Selector1/2 -> Bus Creator/5  "<q>"
  Bus Creator/1 -> AirSensorData/1
  Gain/1 -> ISA Atmosphere Model/1
  AirData/1 -> Bus Selector1/1
  Get Z/1 -> Gain/1
  B747 State/1 -> Bus Selector3/1
  Bus Selector1/3 -> Bus Creator/6  "<alpha>"
  Bus Selector1/4 -> Bus Creator/7  "<beta>"
  Bus Selector1/5 -> Bus Creator/8  "<Ma>"
  Gain1/1 -> Bus Creator/9  "ias"
  ISA Atmosphere Model/1 -> Temperature Conversion/1  "OAT"
  ISA Atmosphere Model/2 -> Speed of Sound/1
  ISA Atmosphere Model/3 -> Bus Creator/2  "static"
  ISA Atmosphere Model/4 -> Bus Creator/3, Rho/1  "rho"

== system simModel2020/PlantModel/B747 Dynamics动力学参数计算 ==
  Wind_e : Inport
  CtrlSurfaces : Inport  Port=2
  Rho : Inport  Port=3
  Speed of Sound : Inport  Port=4
  Deviation On : Inport  Port=5
  6DOF Equations of Motion运动学方程 : Subsystem  VariantControl=use_aerospace_blocks == 1
  Bus Selector : BusSelector  OutputSignals=FQ
  Forces and Moments动力学计算 : Subsystem
  B747 State : Outport
  AirData : Outport  Port=2
  Engine : Outport  Port=3
  Wind : Outport  Port=4
  wires:
  6DOF Equations of Motion运动学方程/1(B747 State) -> Forces and Moments动力学计算/1(B747 State), B747 State/1
  CtrlSurfaces/1 -> Forces and Moments动力学计算/4(CtrlSurfaces)
  Rho/1 -> Forces and Moments动力学计算/3(Rho)
  Wind_e/1 -> Forces and Moments动力学计算/2(Wind_e)
  Forces and Moments动力学计算/1(AirData) -> AirData/1
  Forces and Moments动力学计算/2(FM_b) -> 6DOF Equations of Motion运动学方程/1(FM_b)
  Forces and Moments动力学计算/3(Engine) -> Engine/1, Bus Selector/1
  Speed of Sound/1 -> Forces and Moments动力学计算/5(Speed of Sound)
  Deviation On/1 -> Forces and Moments动力学计算/6(Deviation On), 6DOF Equations of Motion运动学方程/4(Deviation On)
  Bus Selector/1 -> 6DOF Equations of Motion运动学方程/2(oil Q)  "<FQ>"
  Forces and Moments动力学计算/4(IsGround) -> 6DOF Equations of Motion运动学方程/3(IsGround)
  Forces and Moments动力学计算/5(Wind) -> Wind/1

== system simModel2020/PlantModel/FlightSwitchModel ==
  CtrlCmds : Inport  SampleTime=B747.sampleTime
  Add : Sum
  Gain : Gain
  If Action Subsystem : Subsystem  TreatAsAtomicUnit=on
  If Action Subsystem1 : Subsystem  TreatAsAtomicUnit=on
  If Action Subsystem2 : Subsystem  TreatAsAtomicUnit=on
  Manually piloted aircraft : Subsystem
  Multiport Switch : MultiPortSwitch  DataPortOrder=Zero-based contiguous  zeroidx=on  SaturateOnIntegerOverflow=off  InputSameDT=off
  Switch Case : SwitchCase  CaseConditions={0,1,2}  ShowDefaultCase=off
  SwitchFlightMode : Constant  Value=0
  ctrlcmds : Outport
  wires:
  Multiport Switch/1 -> ctrlcmds/1
  Add/1 -> If Action Subsystem2/1(CtrlCmds)
  If Action Subsystem1/1(Out1) -> Multiport Switch/2
  If Action Subsystem2/1(Out1) -> Multiport Switch/3
  Switch Case/3 -> If Action Subsystem/Action
  Switch Case/1 -> If Action Subsystem1/Action
  Manually piloted aircraft/1(Out1) -> If Action Subsystem/1(In1), Gain/1
  CtrlCmds/1 -> If Action Subsystem1/1(CtrlCmds), Add/1
  SwitchFlightMode/1 -> Multiport Switch/1, Switch Case/1
  Switch Case/2 -> If Action Subsystem2/Action
  If Action Subsystem/1(Out1) -> Multiport Switch/4
  Gain/1 -> Add/2

== system simModel2020/PlantModel/Sensor Model ==
  B747 State : Inport
  Wind : Inport  Port=2
  AirSensorData : Inport  Port=3
  Engine : Inport  Port=4
  CtrlSurfaces : Inport  Port=5
  Assemble GPS and State Data : Subsystem
  Noise Model : Subsystem  TreatAsAtomicUnit=on
  SensorData : Outport
  wires:
  Noise Model/1(SensorData) -> SensorData/1
  AirSensorData/1 -> Assemble GPS and State Data/1(AirSensorData)
  CtrlSurfaces/1 -> Assemble GPS and State Data/3(CtrlSurfaces)
  B747 State/1 -> Assemble GPS and State Data/2(B747 State)
  Assemble GPS and State Data/1(B747 StateBus) -> Noise Model/1(B747 State)  "B747 State"
  Engine/1 -> Assemble GPS and State Data/4(Engine)
  Wind/1 -> Assemble GPS and State Data/5(Wind)

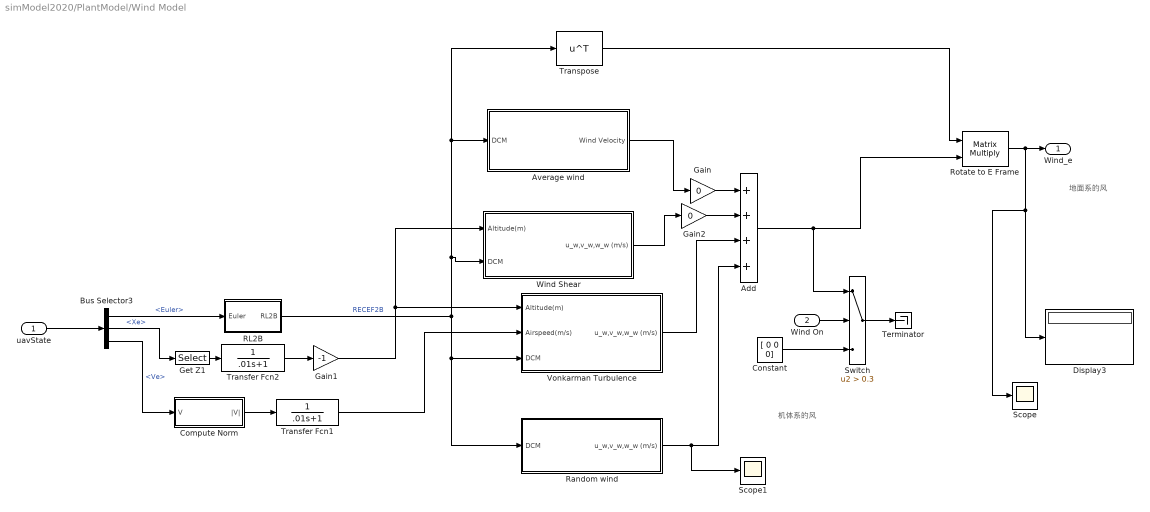
== system simModel2020/PlantModel/Wind Model ==
  note: 地面系的风
  note: 机体系的风
  uavState : Inport
  Wind On : Inport  Port=2
  " Compute Norm" : Subsystem
  Add : Sum  Inputs=4
  Average wind : Subsystem  mask{Vwind=10, Wdeg=0}
      mask prompts: Vwind "Wind speed at altitude (m/s):"; Wdeg "Wind direction at altitude (degrees clockwise from north):"
      mask DialogControl DescGroupVar Prompt: Average wind
      mask DialogControl DescTextVar Prompt: Transform horizontal wind (north and east components) into body coordinates given wind speed, wind direction and direction cosine matrix (DCM).
  Bus Selector3 : BusSelector  OutputSignals=Euler,Xe,Ve
  Constant : Constant  Value=[ 0 0 0]
      settings: AttributesFormatString=%<Value>
  Display3 : Display
  Gain : Gain  Gain=0
  Gain1 : Gain  Gain=-1
      settings: AttributesFormatString=Z to Alt
  Gain2 : Gain  Gain=0
  Get Z1 : Selector  InputPortWidth=3  IndexOptions=Index vector (dialog)  Indices=[3]  OutputSizes=[(-2)]
  RL2B : Subsystem
  Random wind : Subsystem  mask{mu=[1 1 1], sigma=[5 5 2]}
      mask prompts: mu "The mean of random winds:"; sigma "Standard deviation of random wind"
      mask DialogControl DescGroupVar Prompt: Random wind
  Rotate to E Frame : Product  Multiplication=Matrix(*)
  Scope : Scope
  Scope1 : Scope
  Switch : Switch  Criteria=u2 > Threshold  Threshold=0.3  SaturateOnIntegerOverflow=off  InputSameDT=off
  Terminator : Terminator
  Transfer Fcn1 : TransferFcn  Denominator=[.01 1]
  Transfer Fcn2 : TransferFcn  Denominator=[.01 1]
  Transpose : Math  Operator=transpose  SignedPower=on
  Vonkarman Turbulence : Subsystem  mask{W20=1, Wdeg=0, TurbProb=10^-2—Light, L_high=762, ts=B747.sampleTime, Seed=[23341 23341 23341], T_on=on}
      mask prompts: W20 "Wind speed at 6m defines the low-altitude intensity(m/s)"; Wdeg "Wind direction at 6m (degrees clockwise from north):"; TurbProb "Probability of exceedance of high-altitude intensity:"; L_high "Scale length at medium/high altitudes (m):"; ts "Band limited noise sample time (sec):"; Seed "Noise seeds [ug vg wg ]:"; T_on "Turbulence on"
      mask init:
      | h_vec = [.5 1.75 3.75 7.5 15 25 35 45 55 65 75 80]*1000;% feet
      | sigma_vec(1,:) = [3.2 2.2 1.5 zeros(1,9)]; % ft/sec
      | sigma_vec(2,:) = [4.2 3.6 3.3 1.6 zeros(1,8)];
      | sigma_vec(3,:) = [6.6 6.9 7.4 6.7 4.6 2.7 0.4 zeros(1,5)];
      | sigma_vec(4,:) = [8.6 9.6 10.6 10.1 8.0 6.6 5.0 4.2 2.7 zeros(1,3)];
      | sigma_vec(5,:) = [11.8 13.0 16.0 15.1 11.6 9.7 8.1 8.2 7.9 4.9 3.2 2.1];
      | sigma_vec(6,:) = [15.6 17.6 23.0 23.6 22.1 20.0 16.0 15.1 12.1 7.9 6.2 5.1];
      | sigma_vec(7,:) = [18.7 21.5 28.4 30.2 30.7 31.0 25.2 23.1 17.5 10.7 8.4 7.2];
      | max_height_low = 1000;
      | min_height_high = 2000;
      mask TypeOptions TurbProb: 2*10^-1 | 10^-1 | 10^-2—Light | 10^-3—Moderate | 10^-4 | 10^-5—Severe | 10^-6
      mask DialogControl DescGroupVar Prompt: Von Karman Wind Turbulence Model
      mask DialogControl DescTextVar Prompt: Generate continuous wind turbulence
  Wind Shear : Subsystem  mask{phase=Category C -Terminal Flight Phase, W_20=10, Wdeg=0}
      mask prompts: phase "Flight phase:"; W_20 "Wind speed at 6 m altitude (m/s):"; Wdeg "Wind direction at 6 m altitude (degrees clockwise from north):"
      mask init:
      | if phase == 1
      | 	z0 = 0.15;
      | else
      | 	z0=2.0;
      | end
      mask TypeOptions phase: Category C -Terminal Flight Phase | Other
      mask DialogControl DescGroupVar Prompt: Wind Shear Model
      mask DialogControl DescTextVar Prompt: Calculate the wind shear from conditions measured at a height of 6 meters (20 feet) above the ground.
  Wind_e : Outport
  wires:
  Bus Selector3/2 -> Get Z1/1  "<Xe>"
  " Compute Norm"/1(|V|) -> Transfer Fcn1/1
  Bus Selector3/1 -> RL2B/1(Euler)  "<Euler>"
  Constant/1 -> Switch/3
  Transfer Fcn2/1 -> Gain1/1
  Bus Selector3/3 -> " Compute Norm"/1(V)  "<Ve>"
  RL2B/1(RL2B) -> Wind Shear/2(DCM), Average wind/1(DCM), Transpose/1, Random wind/1(DCM), Vonkarman Turbulence/3(DCM)  "RECEF2B"
  Transpose/1 -> Rotate to E Frame/1
  Rotate to E Frame/1 -> Scope/1, Display3/1, Wind_e/1
  uavState/1 -> Bus Selector3/1
  Get Z1/1 -> Transfer Fcn2/1
  Wind On/1 -> Switch/2
  Transfer Fcn1/1 -> Vonkarman Turbulence/2(Airspeed(m/s))
  Average wind/1(Wind Velocity) -> Gain/1
  Wind Shear/1(u_w,v_w,w_w (m/s)) -> Gain2/1
  Vonkarman Turbulence/1(u_w,v_w,w_w (m/s)) -> Add/3
  Random wind/1(u_w,v_w,w_w (m/s)) -> Scope1/1, Add/4
  Gain1/1 -> Wind Shear/1(Altitude(m)), Vonkarman Turbulence/1(Altitude(m))
  Add/1 -> Switch/1, Rotate to E Frame/2
  Switch/1 -> Terminator/1
  Gain/1 -> Add/1
  Gain2/1 -> Add/2

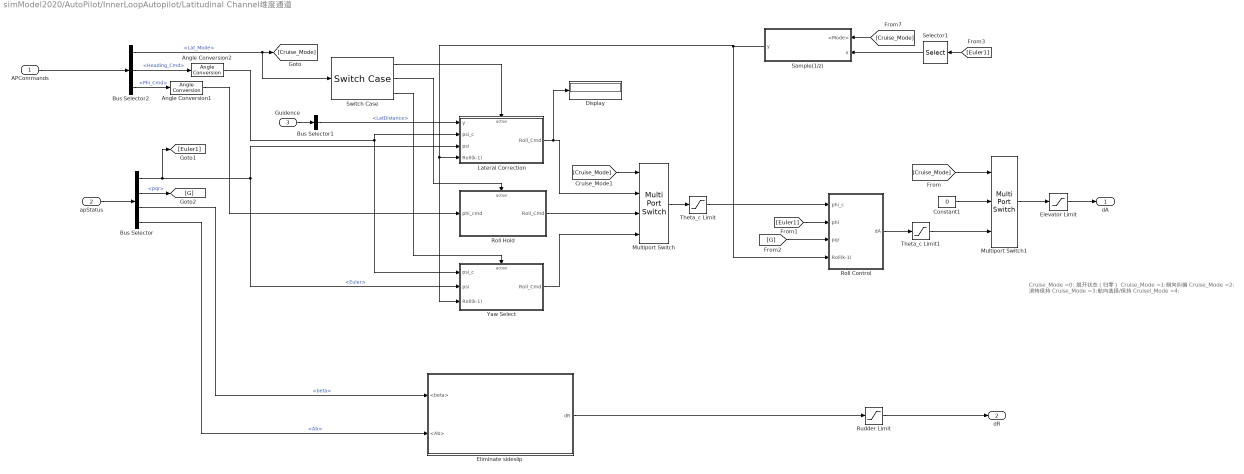
== system simModel2020/AutoPilot/InnerLoopAutopilot/Latitudinal Channel维度通道 ==
  note: Cruise_Mode =0: 脱开状态（归零）
      | Cruise_Mode =1:侧向纠偏
      | Cruise_Mode =2: 滚转保持
      | Cruise_Mode =3:航向选择/保持
      | Cruisel_Mode =4:
  APCommands : Inport
  apStatus : Inport  Port=2
  Guidence : Inport  Port=3
  Angle Conversion1 : aerolibconvert2/Angle Conversion  IU=deg  OU=rad
  Angle Conversion2 : aerolibconvert2/Angle Conversion  IU=deg  OU=rad
  Bus Selector : BusSelector  OutputSignals=Euler,pqr,beta,Ab
  Bus Selector1 : BusSelector  OutputSignals=LatDistance
  Bus Selector2 : BusSelector  OutputSignals=Lat_Mode,Heading_Cmd,Phi_Cmd
  Constant1 : Constant  Value=0
  Display : Display
  Elevator Limit : Saturate  UpperLimit=control.daLimit  LowerLimit=-control.daLimit
      settings: AttributesFormatString="[%<LowerLimit>  %<UpperLimit>]"
  Eliminate sideslip : Subsystem
  Lateral Correction : Subsystem  TreatAsAtomicUnit=on
  Multiport Switch : MultiPortSwitch  DiagnosticForDefault=None  SaturateOnIntegerOverflow=off  InputSameDT=off
  Multiport Switch1 : MultiPortSwitch  DataPortOrder=Zero-based contiguous  Inputs=2  DiagnosticForDefault=None  zeroidx=on  SaturateOnIntegerOverflow=off  InputSameDT=off
  Roll Control : Subsystem
  Roll Hold : Subsystem  TreatAsAtomicUnit=on
  Rudder Limit : Saturate  UpperLimit=control.drLimit  LowerLimit=-control.drLimit
      settings: AttributesFormatString="[%<LowerLimit>  %<UpperLimit>]"
  Sample(1/z) : Subsystem
  Selector1 : Selector  InputPortWidth=3  IndexOptions=Index vector (dialog)  Indices=[1]  OutputSizes=1
  Switch Case : SwitchCase  CaseConditions={1,2,3}  ShowDefaultCase=off
  Theta_c Limit : Saturate  UpperLimit=control.phi_cLimit  LowerLimit=-control.phi_cLimit
      settings: AttributesFormatString="[%<LowerLimit>  %<UpperLimit>]"
  Theta_c Limit1 : Saturate  UpperLimit=control.daLimit  LowerLimit=-control.daLimit
      settings: AttributesFormatString="[%<LowerLimit>  %<UpperLimit>]"
  Yaw Select : Subsystem  TreatAsAtomicUnit=on
  dA : Outport
  dR : Outport  Port=2
  wires:
  apStatus/1 -> Bus Selector/1
  Bus Selector/2 -> [G]  "<pqr>"
  Bus Selector/3 -> Eliminate sideslip/1(<beta>)  "<beta>"
  Bus Selector/4 -> Eliminate sideslip/2(<Ab>)  "<Ab>"
  APCommands/1 -> Bus Selector2/1
  Bus Selector2/1 -> Switch Case/1, [Cruise_Mode]  "<Lat_Mode>"
  Bus Selector2/2 -> Angle Conversion2/1  "<Heading_Cmd>"
  Bus Selector/1 -> Yaw Select/2(psi), Lateral Correction/3(psi), [Euler1]  "<Euler>"
  Switch Case/1 -> Lateral Correction/Action
  Switch Case/2 -> Roll Hold/Action
  Yaw Select/1(Roll_Cmd) -> Multiport Switch/4
  Lateral Correction/1(Roll_Cmd) -> Display/1, Multiport Switch/2
  Roll Hold/1(Roll_Cmd) -> Multiport Switch/3
  Multiport Switch/1 -> Theta_c Limit/1
  Theta_c Limit/1 -> Roll Control/1(phi_c)
  Roll Control/1(dA) -> Theta_c Limit1/1
  Multiport Switch1/1 -> Elevator Limit/1
  Eliminate sideslip/1(dR) -> Rudder Limit/1
  Constant1/1 -> Multiport Switch1/2
  [Euler1] -> Roll Control/2(phi)
  [G] -> Roll Control/3(pqr)
  Rudder Limit/1 -> dR/1
  [Cruise_Mode] -> Sample(1/z)/1(<Mode>)
  [Euler1] -> Selector1/1
  Selector1/1 -> Sample(1/z)/2(x)
  Sample(1/z)/1(y) -> Yaw Select/3(Roll(k-1)), Lateral Correction/4(Roll(k-1)), Roll Control/4(Roll(k-1))
  Guidence/1 -> Bus Selector1/1
  Angle Conversion2/1 -> Lateral Correction/2(psi_c), Yaw Select/1(psi_c)
  Angle Conversion1/1 -> Roll Hold/1(phi_cmd)
  Theta_c Limit1/1 -> Multiport Switch1/3
  Elevator Limit/1 -> dA/1
  [Cruise_Mode] -> Multiport Switch1/1
  Bus Selector2/3 -> Angle Conversion1/1  "<Phi_Cmd>"
  [Cruise_Mode] -> Multiport Switch/1
  Bus Selector1/1 -> Lateral Correction/1(y)  "<LatDistance>"
  Switch Case/3 -> Yaw Select/Action

== system simModel2020/AutoPilot/InnerLoopAutopilot/Longitudinal Channel经度通道 ==
  StatusBus : Inport
  N1 : Inport  Port=2
  APCommands : Inport  Port=3
  AutoThrottle : Subsystem
  Bus Selector1 : BusSelector  OutputSignals=ias,Euler,Xe,Ve,pqr
  PitchStyle : Subsystem
  dE : Outport
  dT : Outport  Port=2
  wires:
  Bus Selector1/1 -> AutoThrottle/3(<ias>), PitchStyle/1(<ias>)  "<ias>"
  StatusBus/1 -> Bus Selector1/1
  N1/1 -> AutoThrottle/2(N1)
  AutoThrottle/1(dT) -> dT/1
  Bus Selector1/2 -> PitchStyle/2(Euler)  "<Euler>"
  Bus Selector1/3 -> PitchStyle/4(<Xe>)  "<Xe>"
  PitchStyle/1(dE) -> dE/1
  Bus Selector1/4 -> PitchStyle/5(Ve)  "<Ve>"
  APCommands/1 -> PitchStyle/3(APCommands), AutoThrottle/1(APCommands)
  Bus Selector1/5 -> PitchStyle/6(pqr)  "<pqr>"

== system simModel2020/Auto_Pilot_Set/Trajectory/Subsystem ==
  In1 : Inport
  In2 : Inport  Port=2
  Derivative : Derivative
  Gain : Gain  Gain=0.02
  Sum : Sum  Inputs=|++
  Transfer Fcn : TransferFcn  Denominator=[1 1]
  Out1 : Outport
  wires:
  In1/1 -> Transfer Fcn/1
  Sum/1 -> Out1/1
  In2/1 -> Sum/2
  Derivative/1 -> Gain/1
  Gain/1 -> Sum/1
  Transfer Fcn/1 -> Derivative/1

== system simModel2020/Draw Aircraft/DataOut/Subsystem ==
  <Wind> : Inport
  Add1 : Sum  Inputs=+++
  Hermitian : Math  Operator=square
  Hermitian1 : Math  Operator=square
  Hermitian2 : Math  Operator=square
  Selector3 : Selector  InputPortWidth=3  IndexOptions=Index vector (dialog)  Indices=[1]  OutputSizes=1
  Selector4 : Selector  InputPortWidth=3  IndexOptions=Index vector (dialog)  Indices=[3]  OutputSizes=1
  Selector5 : Selector  InputPortWidth=3  IndexOptions=Index vector (dialog)  Indices=[2]  OutputSizes=1
  Sqrt : Sqrt
  Out1 : Outport
  Out2 : Outport  Port=2
  Out3 : Outport  Port=3
  Out4 : Outport  Port=4
  wires:
  Add1/1 -> Sqrt/1
  Hermitian2/1 -> Add1/3
  Selector5/1 -> Out2/1, Hermitian1/1
  <Wind>/1 -> Selector4/1, Selector3/1, Selector5/1
  Selector4/1 -> Out3/1, Hermitian2/1
  Sqrt/1 -> Out4/1
  Hermitian/1 -> Add1/1
  Selector3/1 -> Out1/1, Hermitian/1
  Hermitian1/1 -> Add1/2

== system simModel2020/Draw Aircraft/FlightGear/Angle Conversion ==
  in : Inport
  Angle Conversion : aerolibconvert2/Angle Conversion  IU=deg  OU=rad
  out : Outport
  wires:
  in/1 -> Angle Conversion/1
  Angle Conversion/1 -> out/1

== system simModel2020/Draw Aircraft/FlightGear/Angle Conversion1 ==
  in : Inport
  Angle Conversion : aerolibconvert2/Angle Conversion  IU=deg  OU=rad
  out : Outport
  wires:
  Angle Conversion/1 -> out/1
  in/1 -> Angle Conversion/1

== system simModel2020/PlantModel/Actuator Model/Linear Second Order Actuators ==
  Ac_dem : Inport
  2*zeta * wn : Gain  Gain=2.0 * z_fin* wn_fin  SaturateOnIntegerOverflow=on  OutDataTypeStr=Inherit: Same as input  ParamDataTypeStr=Inherit: Same as input
  "Integrator, Second-Order" : SecondOrderIntegrator  ICX=fin_act_0  UpperLimitX=1  LowerLimitX=0  ICDXDT=fin_act_vel
  Sum2 : Sum  Inputs=|+-  InputSameDT=on  SaturateOnIntegerOverflow=on  OutDataTypeStr=Inherit: Same as first input
  Sum3 : Sum  Inputs=|+-  InputSameDT=on  SaturateOnIntegerOverflow=on  OutDataTypeStr=Inherit: Same as first input
  wn^2 : Gain  Gain=wn_fin* wn_fin  SaturateOnIntegerOverflow=on  OutDataTypeStr=Inherit: Same as input  ParamDataTypeStr=Inherit: Same as input
  Ac_ac : Outport  InitialOutput=0
  wires:
  "Integrator, Second-Order"/1 -> Ac_ac/1, Sum3/2
  wn^2/1 -> Sum2/1
  Sum2/1 -> "Integrator, Second-Order"/1
  2*zeta * wn/1 -> Sum2/2
  Ac_dem/1 -> Sum3/1
  Sum3/1 -> wn^2/1
  "Integrator, Second-Order"/2 -> 2*zeta * wn/1

== system simModel2020/PlantModel/Actuator Model/Linear Second-Order Actuator1 ==
  Ac_dem : Inport
  2*zeta * wn : Gain  Gain=2.0 * z_fin* wn_fin  SaturateOnIntegerOverflow=on  OutDataTypeStr=Inherit: Same as input  ParamDataTypeStr=Inherit: Same as input
  "Integrator, Second-Order" : SecondOrderIntegrator  ICX=fin_act_0  UpperLimitX=1  LowerLimitX=0  ICDXDT=fin_act_vel
  Sum2 : Sum  Inputs=|+-  InputSameDT=on  SaturateOnIntegerOverflow=on  OutDataTypeStr=Inherit: Same as first input
  Sum3 : Sum  Inputs=|+-  InputSameDT=on  SaturateOnIntegerOverflow=on  OutDataTypeStr=Inherit: Same as first input
  wn^2 : Gain  Gain=wn_fin* wn_fin  SaturateOnIntegerOverflow=on  OutDataTypeStr=Inherit: Same as input  ParamDataTypeStr=Inherit: Same as input
  Ac_ac : Outport  InitialOutput=0
  wires:
  "Integrator, Second-Order"/1 -> Ac_ac/1, Sum3/2
  wn^2/1 -> Sum2/1
  Sum2/1 -> "Integrator, Second-Order"/1
  2*zeta * wn/1 -> Sum2/2
  Ac_dem/1 -> Sum3/1
  Sum3/1 -> wn^2/1
  "Integrator, Second-Order"/2 -> 2*zeta * wn/1

== system simModel2020/PlantModel/Actuator Model/Linear Second-Order Actuator2 ==
  Ac_dem : Inport
  2*zeta * wn : Gain  Gain=2.0 * z_fin* wn_fin  SaturateOnIntegerOverflow=on  OutDataTypeStr=Inherit: Same as input  ParamDataTypeStr=Inherit: Same as input
  "Integrator, Second-Order" : SecondOrderIntegrator  ICX=fin_act_0  UpperLimitX=1  LowerLimitX=0  ICDXDT=fin_act_vel
  Sum2 : Sum  Inputs=|+-  InputSameDT=on  SaturateOnIntegerOverflow=on  OutDataTypeStr=Inherit: Same as first input
  Sum3 : Sum  Inputs=|+-  InputSameDT=on  SaturateOnIntegerOverflow=on  OutDataTypeStr=Inherit: Same as first input
  wn^2 : Gain  Gain=wn_fin* wn_fin  SaturateOnIntegerOverflow=on  OutDataTypeStr=Inherit: Same as input  ParamDataTypeStr=Inherit: Same as input
  Ac_ac : Outport  InitialOutput=0
  wires:
  "Integrator, Second-Order"/1 -> Ac_ac/1, Sum3/2
  wn^2/1 -> Sum2/1
  Sum2/1 -> "Integrator, Second-Order"/1
  2*zeta * wn/1 -> Sum2/2
  Ac_dem/1 -> Sum3/1
  Sum3/1 -> wn^2/1
  "Integrator, Second-Order"/2 -> 2*zeta * wn/1

== system simModel2020/PlantModel/Actuator Model/Linear Second-Order Actuator3 ==
  Ac_dem : Inport
  2*zeta * wn : Gain  Gain=2.0 * z_fin* wn_fin  SaturateOnIntegerOverflow=on  OutDataTypeStr=Inherit: Same as input  ParamDataTypeStr=Inherit: Same as input
  "Integrator, Second-Order" : SecondOrderIntegrator  ICX=fin_act_0  UpperLimitX=1  LowerLimitX=0  ICDXDT=fin_act_vel
  Sum2 : Sum  Inputs=|+-  InputSameDT=on  SaturateOnIntegerOverflow=on  OutDataTypeStr=Inherit: Same as first input
  Sum3 : Sum  Inputs=|+-  InputSameDT=on  SaturateOnIntegerOverflow=on  OutDataTypeStr=Inherit: Same as first input
  wn^2 : Gain  Gain=wn_fin* wn_fin  SaturateOnIntegerOverflow=on  OutDataTypeStr=Inherit: Same as input  ParamDataTypeStr=Inherit: Same as input
  Ac_ac : Outport  InitialOutput=0
  wires:
  "Integrator, Second-Order"/1 -> Ac_ac/1, Sum3/2
  wn^2/1 -> Sum2/1
  Sum2/1 -> "Integrator, Second-Order"/1
  2*zeta * wn/1 -> Sum2/2
  Ac_dem/1 -> Sum3/1
  Sum3/1 -> wn^2/1
  "Integrator, Second-Order"/2 -> 2*zeta * wn/1
